simulink library "Storage_Type_3_CONF"  (Simulink 8.2)
settings: Solver=ode45  StartTime=0.0  StopTime=10.0  RelTol=1e-3
libraries: carnot x2
settings Model: Creator=lena.frank  LastModifiedBy=drhf

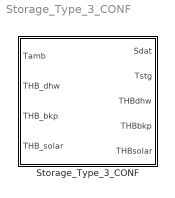
== system Storage_Type_3_CONF ==
  Storage_Type_3_CONF : Subsystem  mask(Storage with 2 heat exchangers and 1 direct port){parameterfile=default_Storage, tini=[10:5:55]}
      mask prompts: parameterfile "Storage parameter set"; tini "initial temperature (vector or scalar) in °C"
      mask help: Predefinded storage with 2 heat exchangers and 1 direct port (for example a bivalent dhw cylinder).
      mask init:
      | % callback to set parameters of model
      | CarnotCallbacks_StorageConf(3,parameterfile);
      mask Help: web(fullfile(path_carnot('help'),'Storage_Type_N.html'),'-helpbrowser')
      mask TypeOptions parameterfile: default_Storage
      mask Display:
      | % user defined picture file
      | picfile = fullfile(path_carnot('intlibsl'), ...
      |         'Storage','Thermal','Storage_Type_3_CONF','parameter_set', ...
      |         'Storage_Type_3_CONF.jpg');
      | 
      | % show public picture
      | plot([36,36,40,50,54,54,50,40,36]/100,[90,50,45,45,50,90,93,93,90]/100, ...
      |     [36,51,40,51,36]/100,[77,77,81,85,85]/100,[36,51,44,51,36]/100, ...
      |     [50,50,55,60,60]/100)
      | 
      | % show internal picture if defined
      | if  ~BlockIsInCarnotLibrary       % if not located in library
      |     if exist(picfile)
      |         image(imread(picfile), [0.25, 0, 0.45, 1])
      |         set_param(gcb, 'BackgroundColor', 'White')
      |     end
      | end

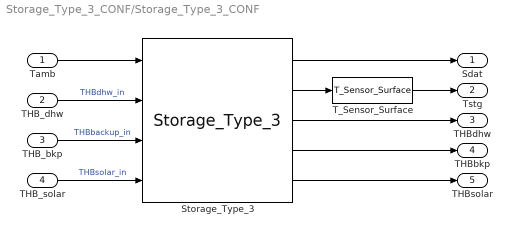
== system Storage_Type_3_CONF/Storage_Type_3_CONF ==
  Tamb : Inport
  THB_dhw : Inport  Port=2
  THB_bkp : Inport  Port=3
  THB_solar : Inport  Port=4
  Storage_Type_3 : carnot/Storage/Thermal/Storage_Type_3  uloss=1  ubot=1  utop=1  cond=1  t0=tini  volume=0.3  dia=0.5  pos=standing cylinder  nconnect=3  nodes=10  mpoints=10
  T_Sensor_Surface : carnot/Control/T_Sensor_Surface  pos="[0.1         0.7]"  tdel=10  t0=tini(1)
  Sdat : Outport
  Tstg : Outport  Port=2
  THBdhw : Outport  Port=3
  THBbkp : Outport  Port=4
  THBsolar : Outport  Port=5
  wires:
  Storage_Type_3/5 -> THBsolar/1
  Storage_Type_3/4 -> THBbkp/1
  Storage_Type_3/3 -> THBdhw/1
  Storage_Type_3/2 -> T_Sensor_Surface/1
  Storage_Type_3/1 -> Sdat/1
  THB_solar/1 -> Storage_Type_3/4  "THBsolar_in"
  THB_bkp/1 -> Storage_Type_3/3  "THBbackup_in"
  THB_dhw/1 -> Storage_Type_3/2  "THBdhw_in"
  Tamb/1 -> Storage_Type_3/1
  T_Sensor_Surface/1 -> Tstg/1
